simulink model "model_pid"  (R2022b)
settings: Solver=ode45  StartTime=0.0  StopTime=1  RelTol=1e-3  EnableMultiTasking=on
values from neighbouring files (symbols this model uses):
  Bm = 1e-04    (= 0.0001)    [loop_estado.m]    (also in loop_pid.m = 5e-08; var_estado.m; var_pid.m = 5e-08)
  g = 1    [loop_pid.m]    (also in sim_pid.m = Gs(i); var_pid.m)
  J = 1e-04    (= 0.0001)    [loop_estado.m]    (also in loop_pid.m = 8e-08; var_estado.m; var_pid.m = 8e-08)
  ka = 0.16    [loop_estado.m]    (also in loop_pid.m = 0.2; var_estado.m; var_pid.m = 0.2)
  kd = 0    [loop_pid.m]    (also in sim_pid.m = KDs(i); var_pid.m)
  kgear = 0.1    [loop_estado.m]    (also in loop_pid.m = 0.01; var_estado.m; var_pid.m = 0.01)
  ki = 250    [loop_pid.m]    (also in var_pid.m)
  kp = 25e3    (= 25000)    [loop_pid.m]    (also in var_pid.m)
  La = 0.0066    [loop_estado.m]    (also in loop_pid.m = 0.002; var_estado.m; var_pid.m = 0.002)
  q = 1    [loop_pid.m]    (also in sim_pid.m = Qs(i); var_pid.m)
  ra = 3.15    [loop_estado.m]    (also in loop_pid.m = 200; var_estado.m; var_pid.m = 200)
  rt = 1    [loop_pid.m]    (also in var_pid.m)
  TL = 0.02    [loop_pid.m]    (also in var_pid.m)
  u_max = 30    [loop_pid.m]    (also in var_pid.m)
  u_min = 0    [loop_pid.m]    (also in var_pid.m)
libraries: slpidlib x1
settings Model: Creator=11802972  LastModifiedBy=andre
settings SolverCC: AlgebraicLoopSolver=TrustRegion
settings DataIOCC: LimitDataPoints=on  SaveFormat=Array  ReturnWorkspaceOutputs=off
settings OptimizationCC: LifeSpan=inf
settings DebuggingCC: UnconnectedInputMsg=warning  UnconnectedOutputMsg=warning  UnconnectedLineMsg=warning  SFUnexpectedBacktrackingDiag=warning  SFNoUnconditionalDefaultTransitionDiag=warning  SFExecutionAtInitializationDiag=none  SFMachineParentedDataDiag=warning  ArithmeticOperatorsInVariantConditions=warning
settings HardwareCC: ProdBitPerPointer=32  ProdBitPerSizeT=32  ProdBitPerPtrDiffT=32  ProdLargestAtomicFloat=None  ProdIntDivRoundTo=Undefined  ProdEndianess=Unspecified  ProdWordSize=32  ProdHWDeviceType=32-bit Generic
settings ModelReferenceCC: PropagateSignalLabelsOutOfModel=off
settings SFSimCC: SimUseLocalCustomCode=off  CustomCodeUndefinedFunction=UseInterfaceOnly
settings RTWCC: RTWUseLocalCustomCode=off
settings CodeAppCC: StateflowObjectComments=on
settings GRTTargetCC: TargetLangStandard=C89/C90 (ANSI)
settings ConfigComp: CovMetricSettings=dw  CovSaveCumulativeToWorkspaceVar=on  CovSaveSingleToWorkspaceVar=on  CovExternalEMLEnable=off

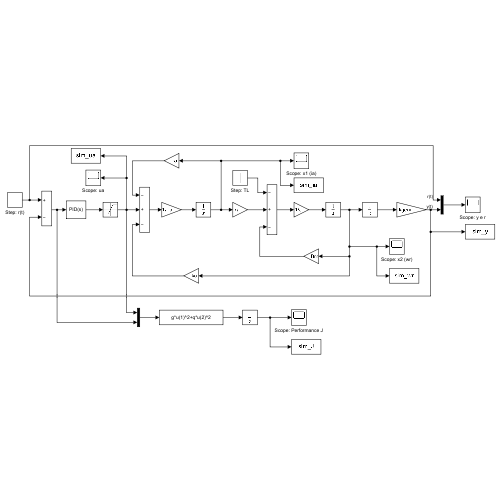
[thumbnail: Simulink's stored preview of the top-level diagram]
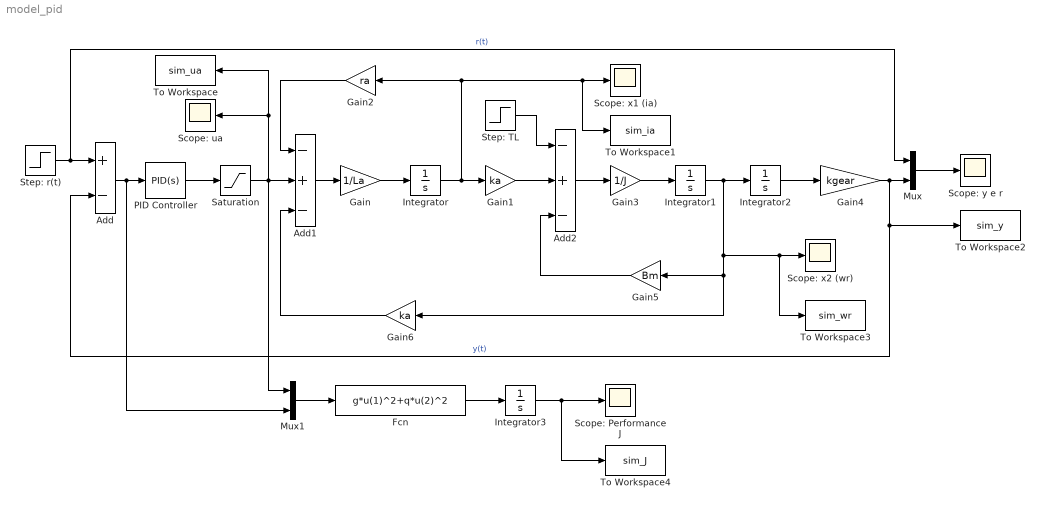
== system model_pid ==
  Add : Sum  Inputs=+-
  Add1 : Sum  Inputs=-+-
  Add2 : Sum  Inputs=-+-
  Fcn : Fcn  Expr=g*u(1)^2+q*u(2)^2
  Gain : Gain  Gain=1/La
  Gain1 : Gain  Gain=ka
  Gain2 : Gain  Gain=ra
  Gain3 : Gain  Gain=1/J
  Gain4 : Gain  Gain=kgear
  Gain5 : Gain  Gain=Bm
  Gain6 : Gain  Gain=ka
  Integrator{,1..3} (4 alike) : Integrator
  Mux : Mux  Inputs=2
  Mux1 : Mux  Inputs=2
  PID Controller : slpidlib/PID Controller  Controller=PID  Form=Parallel  TimeDomain=Continuous-time  UseExternalTs=off  SampleTime=-1  IntegratorMethod=Forward Euler  FilterMethod=Forward Euler  ControllerParametersSource=internal  P=kp  I=ki  UseKiTs=off  D=kd  N=100  UseFilter=on  TunerSelectOption=Transfer Function Based (PID Tuner App)  InitialConditionSource=internal  InitialConditionForIntegrator=0  InitialConditionForFilter=0  DifferentiatorICPrevScaledInput=0  ExternalReset=none  TrackingMode=off  Kt=1  LimitOutput=off  SatLimitsSource=internal  UpperSaturationLimit=inf  LowerSaturationLimit=-inf  LinearizeAsGain=on  AntiWindupMode=none  Kb=1  LimitIntegrator=off  UpperIntegratorSaturationLimit=inf  LowerIntegratorSaturationLimit=-inf  POutMin=[]  POutMax=[]  IOutMin=[]  IOutMax=[]  DOutMin=[]  DOutMax=[]  NOutMin=[]  NOutMax=[]  SumOutMin=[]  SumOutMax=[]  SaturationOutMin=[]  SaturationOutMax=[]  PParamMin=[]  PParamMax=[]  IParamMin=[]  IParamMax=[]  DParamMin=[]  DParamMax=[]  NParamMin=[]  NParamMax=[]  KbParamMin=[]  KbParamMax=[]  KtParamMin=[]  KtParamMax=[]  KbOutMin=[]  KbOutMax=[]  KtOutMin=[]  KtOutMax=[]  IntegratorOutMin=[]  IntegratorOutMax=[]  FilterOutMin=[]  FilterOutMax=[]  SumI1OutMin=[]  SumI1OutMax=[]  SumI2OutMin=[]  SumI2OutMax=[]  SumI3OutMin=[]  SumI3OutMax=[]  SumI4OutMin=[]  SumI4OutMax=[]  SumDOutMin=[]  SumDOutMax=[]  DifferentiatorOutMin=[]  DifferentiatorOutMax=[]  FilterDiffOutCoefMin=[]  FilterDiffOutCoefMax=[]  ReciprocalOutMin=[]  ReciprocalOutMax=[]  SumDenOutMin=[]  SumDenOutMax=[]  SumNumOutMin=[]  SumNumOutMax=[]  DivideOutMin=[]  DivideOutMax=[]  UdiffTsProdOutMin=[]  UdiffTsProdOutMax=[]  NTsProdOutMin=[]  NTsProdOutMax=[]  UintegralTsProdOutMin=[]  UintegralTsProdOutMax=[]  UngainTsProdOutMin=[]  UngainTsProdOutMax=[]  ClampingZeroOutDataTypeStr=Inherit: Inherit via back propagation  ClampingZeroOutMin=[]  ClampingZeroOutMax=[]  FilterDenConstantOutDataTypeStr=Inherit: Inherit via back propagation  FilterDenConstantOutMin=[]  FilterDenConstantOutMax=[]  PCopyOutDataTypeStr=Inherit: Inherit via back propagation  PCopyOutMin=[]  PCopyOutMax=[]  NCopyOutDataTypeStr=Inherit: Inherit via back propagation  NCopyOutMin=[]  NCopyOutMax=[]  IntegratorContinuousStateAttributes=''  IntegratorStateMustResolveToSignalObject=off  IntegratorRTWStateStorageClass=Auto  FilterContinuousStateAttributes=''  FilterStateMustResolveToSignalObject=off  FilterRTWStateStorageClass=Auto  ParallelPVariant=InternalParameters  IdealPVariant=Disabled  IVariant=InternalParameters  DVariant=InternalParameters  IntegratorVariant=Continuous  SatVariant=Disabled  AWVariant=Passthrough  PCopyVariant=Disabled  TRVariant=Disabled  FdbkBlocksVariant=Forward  IdealPFdbkVariant=Disabled  SatFdbkVariant=Disabled  DerivativeFilterVariant=ContFilter  NVariant=InternalParameters  NCopyVariant=Disabled  FilterICVariant=InternalICsFilter  IntegratorICVariant=InternalICs  ExternalResetVariant=Disabled  TRSumVariant=Passthrough  SumFdbkVariant=Disabled  SumVariant=Sum_PID  TsampFilterVariant=InternalTs  TsampNgainVariant=Passthrough  TsampIntegralVariant=Passthrough  ExternalSaturationOutDataTypeStr=Inherit: Same as second input
  Saturation : Saturate  UpperLimit=u_max  LowerLimit=u_min
  Scope: Performance J : Scope
  Scope: ua : Scope
  Scope: x1 (ia) : Scope
  Scope: x2 (wr) : Scope
  Scope: y e r : Scope
  Step: TL : Step  Time=0.8  After=TL  SampleTime=0
  Step: r(t) : Step  Time=0  After=rt  SampleTime=0
  To Workspace : ToWorkspace  VariableName=sim_ua  SaveFormat=Timeseries  SampleTime=-1
  To Workspace1 : ToWorkspace  VariableName=sim_ia  SaveFormat=Timeseries  SampleTime=-1
  To Workspace2 : ToWorkspace  VariableName=sim_y  SaveFormat=Timeseries  SampleTime=-1
  To Workspace3 : ToWorkspace  VariableName=sim_wr  SaveFormat=Timeseries  SampleTime=-1
  To Workspace4 : ToWorkspace  VariableName=sim_J  SaveFormat=Timeseries  SampleTime=-1
  wires:
  Step: r(t)/1 -> Mux/1, Add/1  "r(t)"
  Add/1 -> Mux1/2, PID Controller/1
  PID Controller/1 -> Saturation/1
  Saturation/1 -> To Workspace/1, Scope: ua/1, Mux1/1, Add1/2
  Add1/1 -> Gain/1
  Gain/1 -> Integrator/1
  Integrator/1 -> Gain2/1, To Workspace1/1, Scope: x1 (ia)/1, Gain1/1
  Gain2/1 -> Add1/1
  Gain1/1 -> Add2/2
  Step: TL/1 -> Add2/1
  Add2/1 -> Gain3/1
  Gain3/1 -> Integrator1/1
  Integrator1/1 -> Gain6/1, Gain5/1, To Workspace3/1, Scope: x2 (wr)/1, Integrator2/1
  Integrator2/1 -> Gain4/1
  Gain4/1 -> To Workspace2/1, Add/2, Mux/2  "y(t)"
  Mux/1 -> Scope: y e r/1
  Gain5/1 -> Add2/3
  Gain6/1 -> Add1/3
  Mux1/1 -> Fcn/1
  Fcn/1 -> Integrator3/1
  Integrator3/1 -> To Workspace4/1, Scope: Performance J/1
